simulink model "momentumBasedFlight"  (R2021b)
settings: Solver=VariableStepAuto  StartTime=0.0  StopTime=Config.simulationTime  RelTol=1e-3
InitFcn:
  | cd(fileparts(which(bdroot)));
  | initMomentumBasedFlight;
StopFcn:
  | cd(fileparts(which(bdroot)));
  | stopMomentumBasedFlight;
undefined symbols (not defined in the file or in its folder): aero_config, biasVectorConstraint_feet, Config, ConstraintMatrix_feet, DiscIntNeverNeededParam, frameNames, Frames
libraries: WBToolboxLibrary x104, momentum_flight_control_sublib x4, thrust_estimation_sublib x1, jets_control x1
(part 3 of 3)

== system momentumBasedFlight/FLIGHT CONTROLLER (CORE) V3.0/Flight Controller RAL-HUMANOIDS V3.0/Momentum Control for Flying/QP Solver and Integrate Contact Forces Derivative ==
  HessianMatrixQP : Inport
  gVectorQP : Inport  Port=2
  lowerBoundQP : Inport  Port=3
  upperBoundQP : Inport  Port=4
  stateMachineQuantities : Inport  Port=5
  systemState : Inport  Port=6
  dynamics : Inport  Port=7
  Bus Selector1 : BusSelector  OutputSignals=feetContactIsActive
  Bus Selector2 : BusSelector  OutputSignals=contactForces
  Integrate the Contact Forces Derivative : Subsystem
  QP momentumControl : Subsystem
  contactForces_star : Outport  VectorParamsAs1DForOutWhenUnconnected=off
  jetsIntensitiesDot_star : Outport  Port=2  VectorParamsAs1DForOutWhenUnconnected=off
  jointVel_star : Outport  Port=3  VectorParamsAs1DForOutWhenUnconnected=off
  tag scope: contactForces_star=global, exitFlagQP_momentumControl=global, jetsIntensitiesDot_star=global, jointVel_star=global
  wires:
  systemState/1 -> Bus Selector2/1
  Bus Selector2/1 -> Integrate the Contact Forces Derivative/2(contactForces)  "<contactForces>"
  Bus Selector1/1 -> Integrate the Contact Forces Derivative/4(feetContactIsActive), QP momentumControl/5(feetContactIsActive)  "<feetContactIsActive>"
  QP momentumControl/3(jointVel_star) -> jointVel_star/1, [jointVel_star]
  QP momentumControl/1(jetsIntensitiesDot_star) -> jetsIntensitiesDot_star/1, [jetsIntensitiesDot_star]
  HessianMatrixQP/1 -> QP momentumControl/1(HessianMatrixQP)
  stateMachineQuantities/1 -> Bus Selector1/1
  gVectorQP/1 -> QP momentumControl/2(gVectorQP)
  QP momentumControl/4(exitFlagQP_momentumControl) -> [exitFlagQP_momentumControl]
  upperBoundQP/1 -> QP momentumControl/4(upperBoundQP)
  lowerBoundQP/1 -> QP momentumControl/3(lowerBoundQP)
  Integrate the Contact Forces Derivative/1(contactForces_star) -> [contactForces_star], contactForces_star/1
  QP momentumControl/2(contactForcesDot_star) -> Integrate the Contact Forces Derivative/1(contactForcesDot_star)
  dynamics/1 -> Integrate the Contact Forces Derivative/3(dynamics)

== system momentumBasedFlight/FLOATING BASE ESTIMATOR/Compute base to fixed link transform/LFoot to base link transform /neck transform ==
  neck port : Inport
  Constant : Constant  Value=zeros(3,1)
  Gain : Gain  Gain=pi/180
  Selector1 : Selector  InputPortWidth=Ports.NECK_POS_PORT_SIZE  IndexOptions=Index vector (dialog)  Indices=[1:3]  OutputSizes=1
  Switch : Switch  Criteria=u2 > Threshold
  USE_IMU4EST_BASE1 : Constant  Value=Config.CORRECT_NECK_IMU
  neck position : Outport  VectorParamsAs1DForOutWhenUnconnected=off
  wires:
  neck port/1 -> Gain/1
  USE_IMU4EST_BASE1/1 -> Switch/2
  Switch/1 -> neck position/1
  Gain/1 -> Selector1/1
  Constant/1 -> Switch/3
  Selector1/1 -> Switch/1  "neck pos"

== system momentumBasedFlight/FLOATING BASE ESTIMATOR/Compute base to fixed link transform/RFoot to base link transform/neck transform ==
  neck port : Inport
  Constant : Constant  Value=zeros(3,1)
  Gain : Gain  Gain=pi/180
  Selector1 : Selector  InputPortWidth=Ports.NECK_POS_PORT_SIZE  IndexOptions=Index vector (dialog)  Indices=[1:3]  OutputSizes=1
  Switch : Switch  Criteria=u2 > Threshold
  USE_IMU4EST_BASE1 : Constant  Value=Config.CORRECT_NECK_IMU
  neck position : Outport  VectorParamsAs1DForOutWhenUnconnected=off
  wires:
  neck port/1 -> Gain/1
  USE_IMU4EST_BASE1/1 -> Switch/2
  Switch/1 -> neck position/1
  Gain/1 -> Selector1/1
  Constant/1 -> Switch/3
  Selector1/1 -> Switch/1  "neck pos"

== system momentumBasedFlight/FLIGHT CONTROLLER (CORE) V3.0/Flight Controller RAL-HUMANOIDS V3.0/Joint Torque Control for Flying/QP torqueControl/QP torqueControl - balancing ==
  H : Inport
  g : Inport  Port=2
  ub : Inport  Port=3
  lb : Inport  Port=4
  AEq : Inport  Port=5
  lbEq : Inport  Port=6
  ubEq : Inport  Port=7
  Enable : EnablePort
  Combine Bounds and Inequalities : MATLAB Function  TreatAsAtomicUnit=on
  MatchSignalSizes : WBToolboxLibrary/Utilities/MatchSignalSizes
      settings: SourceProductName=WholeBodyToolbox
  QP balancing-torqueControl : WBToolboxLibrary/Utilities/QP  lbA=on  ubA=on  lb=off  ub=off  computeObjVal=off  stopIfFails=off
      settings: SourceProductName=WholeBodyToolbox
  QPStatus_balancing : Outport  VectorParamsAs1DForOutWhenUnconnected=off
  QPOutput_balancing : Outport  Port=2  VectorParamsAs1DForOutWhenUnconnected=off
  wires:
  Combine Bounds and Inequalities/3(ubEq_combined) -> QP balancing-torqueControl/5
  Combine Bounds and Inequalities/2(lbEq_combined) -> QP balancing-torqueControl/4
  Combine Bounds and Inequalities/1(AEq_combined) -> QP balancing-torqueControl/3
  ub/1 -> Combine Bounds and Inequalities/5(ub)
  lb/1 -> Combine Bounds and Inequalities/4(lb)
  ubEq/1 -> Combine Bounds and Inequalities/3(ubEq)
  lbEq/1 -> Combine Bounds and Inequalities/2(lbEq)
  AEq/1 -> Combine Bounds and Inequalities/1(AEq)
  g/1 -> QP balancing-torqueControl/2, MatchSignalSizes/1
  H/1 -> QP balancing-torqueControl/1
  QP balancing-torqueControl/1 -> MatchSignalSizes/2
  MatchSignalSizes/1 -> QPOutput_balancing/1
  QP balancing-torqueControl/2 -> QPStatus_balancing/1

== system momentumBasedFlight/FLIGHT CONTROLLER (CORE) V3.0/Flight Controller RAL-HUMANOIDS V3.0/Joint Torque Control for Flying/QP torqueControl/QP torqueControl - flight ==
  H : Inport
  g : Inport  Port=2
  ub : Inport  Port=3
  lb : Inport  Port=4
  Enable : EnablePort
  Constant : Constant  Value=eye(Config.N_DOF)
  MatchSignalSizes : WBToolboxLibrary/Utilities/MatchSignalSizes
      settings: SourceProductName=WholeBodyToolbox
  QP flight-torqueControl : WBToolboxLibrary/Utilities/QP  lbA=on  ubA=on  lb=off  ub=off  computeObjVal=off  stopIfFails=off
      settings: SourceProductName=WholeBodyToolbox
  QPStatus_flight : Outport  VectorParamsAs1DForOutWhenUnconnected=off
  QPOutput_flight : Outport  Port=2  VectorParamsAs1DForOutWhenUnconnected=off
  wires:
  ub/1 -> QP flight-torqueControl/5
  g/1 -> MatchSignalSizes/1, QP flight-torqueControl/2
  H/1 -> QP flight-torqueControl/1
  QP flight-torqueControl/1 -> MatchSignalSizes/2
  MatchSignalSizes/1 -> QPOutput_flight/1
  lb/1 -> QP flight-torqueControl/4
  QP flight-torqueControl/2 -> QPStatus_flight/1
  Constant/1 -> QP flight-torqueControl/3

== system momentumBasedFlight/FLIGHT CONTROLLER (CORE) V3.0/Flight Controller RAL-HUMANOIDS V3.0/Joint Torque Control for Flying/QP torqueControl/Select QP torqueControl Output ==
  QPStatus_balancing : Inport
  QPOutput_balancing : Inport  Port=2
  feetContactIsActive : Inport  Port=3
  QPStatus_flight : Inport  Port=4
  QPOutput_flight : Inport  Port=5
  Demux : Demux  Outputs=[12;Config.N_DOF]
  Switch : Switch  Criteria=u2 > Threshold
  Switch1 : Switch  Criteria=u2 > Threshold
  jointTorques_star : Outport  VectorParamsAs1DForOutWhenUnconnected=off
  exitFlagQP_torqueControl : Outport  Port=2  VectorParamsAs1DForOutWhenUnconnected=off
  contactForces_QP_star : Outport  Port=3  VectorParamsAs1DForOutWhenUnconnected=off
  wires:
  Demux/2 -> Switch1/1
  Demux/1 -> contactForces_QP_star/1
  QPOutput_flight/1 -> Switch1/3
  QPOutput_balancing/1 -> Demux/1
  Switch/1 -> exitFlagQP_torqueControl/1
  QPStatus_flight/1 -> Switch/3
  QPStatus_balancing/1 -> Switch/1
  feetContactIsActive/1 -> Switch/2, Switch1/2
  Switch1/1 -> jointTorques_star/1

== system momentumBasedFlight/FLIGHT CONTROLLER (CORE) V3.0/Flight Controller RAL-HUMANOIDS V3.0/Momentum Control for Flying/QP Solver and Integrate Contact Forces Derivative/Integrate the Contact Forces Derivative ==
  contactForcesDot_star : Inport
  contactForces : Inport  Port=2
  dynamics : Inport  Port=3
  feetContactIsActive : Inport  Port=4
  Bus Selector2 : BusSelector  OutputSignals=M
  Discrete-Time Integrator1 : DiscreteIntegrator  ExternalReset=either  InitialConditionSource=external  InitialCondition=zeros(6,1)  SampleTime=Config.tStep  ICPrevOutput=DiscIntNeverNeededParam  ICPrevScaledInput=DiscIntNeverNeededParam
  Select Integrator Initial Condition : MATLAB Function  TreatAsAtomicUnit=on
  Selector : Selector  NumberOfDimensions=2  InputPortWidth=3  IndexOptions=Index vector (dialog),Index vector (dialog)  Indices=1,1  OutputSizes=1,1
  deadZone : Subsystem
  contactForces_star : Outport  VectorParamsAs1DForOutWhenUnconnected=off
  tag scope: contactForcesDot_star=global
  wires:
  Select Integrator Initial Condition/1(contactForces_0) -> Discrete-Time Integrator1/3
  feetContactIsActive/1 -> Discrete-Time Integrator1/2, Select Integrator Initial Condition/1(feetContactIsActive)
  contactForces/1 -> Select Integrator Initial Condition/2(contactForces)
  deadZone/1(u_cut) -> Discrete-Time Integrator1/1
  contactForcesDot_star/1 -> [contactForcesDot_star], deadZone/1(u)
  Discrete-Time Integrator1/1 -> contactForces_star/1
  dynamics/1 -> Bus Selector2/1
  Bus Selector2/1 -> Selector/1  "<M>"
  Selector/1 -> Select Integrator Initial Condition/3(m)

== system momentumBasedFlight/FLIGHT CONTROLLER (CORE) V3.0/Flight Controller RAL-HUMANOIDS V3.0/Momentum Control for Flying/QP Solver and Integrate Contact Forces Derivative/QP momentumControl ==
  HessianMatrixQP : Inport
  gVectorQP : Inport  Port=2
  lowerBoundQP : Inport  Port=3
  upperBoundQP : Inport  Port=4
  feetContactIsActive : Inport  Port=5
  NOT : Logic  Operator=NOT  IconShape=distinctive  AllPortsSameDT=off  OutDataTypeStr=boolean
  Process QP Inputs Momentum Control : MATLAB Function  TreatAsAtomicUnit=on
  QP momentumControl - balancing : Subsystem  TreatAsAtomicUnit=on
  QP momentumControl - flight : Subsystem  TreatAsAtomicUnit=on
  Select QP momentumControl Output : Subsystem
  jetsIntensitiesDot_star : Outport  VectorParamsAs1DForOutWhenUnconnected=off
  contactForcesDot_star : Outport  Port=2  VectorParamsAs1DForOutWhenUnconnected=off
  jointVel_star : Outport  Port=3  VectorParamsAs1DForOutWhenUnconnected=off
  exitFlagQP_momentumControl : Outport  Port=4  VectorParamsAs1DForOutWhenUnconnected=off
  wires:
  QP momentumControl - flight/2(QPOutput_flight) -> Select QP momentumControl Output/5(QPOutput_flight)
  QP momentumControl - flight/1(QPStatus_flight) -> Select QP momentumControl Output/4(QPStatus_flight)
  QP momentumControl - balancing/2(QPOutput_balancing) -> Select QP momentumControl Output/2(QPOutput_balancing)
  QP momentumControl - balancing/1(QPStatus_balancing) -> Select QP momentumControl Output/1(QPStatus_balancing)
  Select QP momentumControl Output/4(exitFlagQP_momentumControl) -> exitFlagQP_momentumControl/1
  NOT/1 -> QP momentumControl - flight/Enable
  Process QP Inputs Momentum Control/8(lb_flight) -> QP momentumControl - flight/4(lb)
  Process QP Inputs Momentum Control/7(ub_flight) -> QP momentumControl - flight/3(ub)
  Process QP Inputs Momentum Control/4(lb_balancing) -> QP momentumControl - balancing/4(lb)
  Process QP Inputs Momentum Control/3(ub_balancing) -> QP momentumControl - balancing/3(ub)
  Process QP Inputs Momentum Control/6(g_flight) -> QP momentumControl - flight/2(g)
  Process QP Inputs Momentum Control/5(H_flight) -> QP momentumControl - flight/1(H)
  Process QP Inputs Momentum Control/2(g_balancing) -> QP momentumControl - balancing/2(g)
  Process QP Inputs Momentum Control/1(H_balancing) -> QP momentumControl - balancing/1(H)
  Select QP momentumControl Output/2(contactForcesDot_star) -> contactForcesDot_star/1
  Select QP momentumControl Output/3(jointVel_star) -> jointVel_star/1
  Select QP momentumControl Output/1(jetsIntensitiesDot_star) -> jetsIntensitiesDot_star/1
  HessianMatrixQP/1 -> Process QP Inputs Momentum Control/1(HessianMatrixQP)
  upperBoundQP/1 -> Process QP Inputs Momentum Control/4(upperBoundQP)
  feetContactIsActive/1 -> QP momentumControl - balancing/Enable, NOT/1, Select QP momentumControl Output/3(feetContactIsActive)
  lowerBoundQP/1 -> Process QP Inputs Momentum Control/3(lowerBoundQP)
  gVectorQP/1 -> Process QP Inputs Momentum Control/2(gVectorQP)

== system momentumBasedFlight/FLIGHT CONTROLLER (CORE) V3.0/Flight Controller RAL-HUMANOIDS V3.0/Momentum Control for Flying/QP Solver and Integrate Contact Forces Derivative/Integrate the Contact Forces Derivative/deadZone ==
  u : Inport
  Constant : Constant  Value=Config.sat.deadZoneThreshold
  Deadzone Function : MATLAB Function  TreatAsAtomicUnit=on
  u_cut : Outport  VectorParamsAs1DForOutWhenUnconnected=off
  wires:
  Constant/1 -> Deadzone Function/2(thr)
  u/1 -> Deadzone Function/1(u)
  Deadzone Function/1(y) -> u_cut/1

== system momentumBasedFlight/FLIGHT CONTROLLER (CORE) V3.0/Flight Controller RAL-HUMANOIDS V3.0/Momentum Control for Flying/QP Solver and Integrate Contact Forces Derivative/QP momentumControl/QP momentumControl - balancing ==
  H : Inport
  g : Inport  Port=2
  ub : Inport  Port=3
  lb : Inport  Port=4
  Enable : EnablePort
  Constant : Constant  Value=eye(Config.N_DOF + 12 + 4)
  MatchSignalSizes : WBToolboxLibrary/Utilities/MatchSignalSizes
      settings: SourceProductName=WholeBodyToolbox
  QP : WBToolboxLibrary/Utilities/QP  lbA=on  ubA=on  lb=off  ub=off  computeObjVal=off  stopIfFails=off
      settings: SourceProductName=WholeBodyToolbox
  QPStatus_balancing : Outport  VectorParamsAs1DForOutWhenUnconnected=off
  QPOutput_balancing : Outport  Port=2  VectorParamsAs1DForOutWhenUnconnected=off
  wires:
  ub/1 -> QP/5
  QP/1 -> MatchSignalSizes/2
  MatchSignalSizes/1 -> QPOutput_balancing/1
  QP/2 -> QPStatus_balancing/1
  H/1 -> QP/1
  g/1 -> MatchSignalSizes/1, QP/2
  lb/1 -> QP/4
  Constant/1 -> QP/3

== system momentumBasedFlight/FLIGHT CONTROLLER (CORE) V3.0/Flight Controller RAL-HUMANOIDS V3.0/Momentum Control for Flying/QP Solver and Integrate Contact Forces Derivative/QP momentumControl/QP momentumControl - flight ==
  H : Inport
  g : Inport  Port=2
  ub : Inport  Port=3
  lb : Inport  Port=4
  Enable : EnablePort
  Constant : Constant  Value=eye(Config.N_DOF + 4)
  MatchSignalSizes : WBToolboxLibrary/Utilities/MatchSignalSizes
      settings: SourceProductName=WholeBodyToolbox
  QP flight-momentumControl : WBToolboxLibrary/Utilities/QP  lbA=on  ubA=on  lb=off  ub=off  computeObjVal=off  stopIfFails=off
      settings: SourceProductName=WholeBodyToolbox
  QPStatus_flight : Outport  VectorParamsAs1DForOutWhenUnconnected=off
  QPOutput_flight : Outport  Port=2  VectorParamsAs1DForOutWhenUnconnected=off
  wires:
  ub/1 -> QP flight-momentumControl/5
  g/1 -> MatchSignalSizes/1, QP flight-momentumControl/2
  H/1 -> QP flight-momentumControl/1
  QP flight-momentumControl/1 -> MatchSignalSizes/2
  MatchSignalSizes/1 -> QPOutput_flight/1
  lb/1 -> QP flight-momentumControl/4
  QP flight-momentumControl/2 -> QPStatus_flight/1
  Constant/1 -> QP flight-momentumControl/3

== system momentumBasedFlight/FLIGHT CONTROLLER (CORE) V3.0/Flight Controller RAL-HUMANOIDS V3.0/Momentum Control for Flying/QP Solver and Integrate Contact Forces Derivative/QP momentumControl/Select QP momentumControl Output ==
  QPStatus_balancing : Inport
  QPOutput_balancing : Inport  Port=2
  feetContactIsActive : Inport  Port=3
  QPStatus_flight : Inport  Port=4
  QPOutput_flight : Inport  Port=5
  Constant : Constant  Value=zeros(12,1)
  Demux : Demux  Outputs=[4;12;Config.N_DOF]
  Demux1 : Demux  Outputs=[4;Config.N_DOF]
  Switch{,1..3} (4 alike) : Switch  Criteria=u2 > Threshold
  jetsIntensitiesDot_star : Outport  VectorParamsAs1DForOutWhenUnconnected=off
  contactForcesDot_star : Outport  Port=2  VectorParamsAs1DForOutWhenUnconnected=off
  jointVel_star : Outport  Port=3  VectorParamsAs1DForOutWhenUnconnected=off
  exitFlagQP_momentumControl : Outport  Port=4  VectorParamsAs1DForOutWhenUnconnected=off
  wires:
  Demux1/2 -> Switch3/3
  Demux/3 -> Switch3/1
  Constant/1 -> Switch2/3
  Demux/2 -> Switch2/1
  Demux1/1 -> Switch1/3
  Demux/1 -> Switch1/1
  QPOutput_flight/1 -> Demux1/1
  QPOutput_balancing/1 -> Demux/1
  Switch/1 -> exitFlagQP_momentumControl/1
  QPStatus_flight/1 -> Switch/3
  QPStatus_balancing/1 -> Switch/1
  feetContactIsActive/1 -> Switch/2, Switch1/2, Switch2/2, Switch3/2
  Switch3/1 -> jointVel_star/1
  Switch1/1 -> jetsIntensitiesDot_star/1
  Switch2/1 -> contactForcesDot_star/1

== matlab function momentumBasedFlight/Visualizer/Task and Base Frame Kinematics/MATLAB Function3 ==
  data: RPY_Corr output; rollPitchYaw input
function RPY_Corr = correctYawAngleFCN(rollPitchYaw)

    RPY_Corr = correctYawAngle(rollPitchYaw);

end

== matlab function momentumBasedFlight/Visualizer/Task and Base Frame Kinematics/Get RPY from rotation matrix  ==
  data: w_R_b input; rollPitchYaw output
function rollPitchYaw = rollPitchYawFromRotationFCN(w_R_b)

rollPitchYaw = wbc.rollPitchYawFromRotation(w_R_b);

end

== matlab function momentumBasedFlight/FLIGHT CONTROLLER (CORE) V3.0/Estimated or Measured Thrusts/fromPosRPYtoTransfMatrix ==
  data: pos_rpy input; w_H_b output
function w_H_b = fromPosRpyToTransfMatrixFCN(pos_rpy)

    w_H_b = wbc.fromPosRpyToTransfMatrix(pos_rpy);
end

== matlab function momentumBasedFlight/Visualizer/Task and Base Frame Kinematics/Get RPY from rotation matrix ==
  data: w_R_b input; rollPitchYaw output
function rollPitchYaw = rollPitchYawFromRotationFCN(w_R_b)

rollPitchYaw = wbc.rollPitchYawFromRotation(w_R_b);

end

== matlab function momentumBasedFlight/Visualizer/Task and Base Frame Kinematics/Get RPY error norm ==
  data: rot_err input; rotErr_norm output
function rotErr_norm = normFCN(rot_err)

rotErr_norm = norm(rot_err);

end

== matlab function momentumBasedFlight/FLIGHT CONTROLLER (CORE) V3.0/Flight Controller RAL-HUMANOIDS V3.0/Joint Torque Control for Flying/QP torqueControl/Process QP Inputs Torque Control ==
  data: HessianMatrixQP input; H_balancing output; gVectorQP input; InequalityConstrMatrix input; biasVectorInequalityConstr input; g_balancing output; ub_balancing output; lb_balancing output; Aeq_balancing output; lbEq_balancing output; ubEq_balancing output; H_flight output; g_flight output; ub_flight output; lb_flight output; jointTorquesSaturation input; Config parameter
function [H_balancing,g_balancing,ub_balancing,lb_balancing,Aeq_balancing,lbEq_balancing,ubEq_balancing, ...
          H_flight,g_flight,ub_flight,lb_flight] = processQPinputTorqueControlFCN ...
                                                       (HessianMatrixQP,gVectorQP,InequalityConstrMatrix, ...
                                                        biasVectorInequalityConstr,jointTorquesSaturation,Config)   
   
[H_balancing,g_balancing,ub_balancing,lb_balancing,Aeq_balancing,lbEq_balancing,ubEq_balancing, ...
          H_flight,g_flight,ub_flight,lb_flight] = iRonCubLib.processQPinputTorqueControl ...
                                                       (HessianMatrixQP,gVectorQP,InequalityConstrMatrix, ...
                                                        biasVectorInequalityConstr,jointTorquesSaturation,Config);     
end

== matlab function momentumBasedFlight/FLIGHT CONTROLLER (CORE) V3.0/Flight Controller RAL-HUMANOIDS V3.0/Joint Torque Control for Flying/QP torqueControl/QP torqueControl - balancing/Combine Bounds and Inequalities ==
  data: AEq input; AEq_combined output; lbEq input; ubEq input; lb input; ub input; lbEq_combined output; ubEq_combined output
function [AEq_combined,lbEq_combined,ubEq_combined] = combineInputBoundsAndInequalitiesQPFCN(AEq,lbEq,ubEq,lb,ub)

   [AEq_combined,lbEq_combined,ubEq_combined] = iRonCubLib.combineInputBoundsAndInequalitiesQP(AEq,lbEq,ubEq,lb,ub);
end

== matlab function momentumBasedFlight/Visualizer/Task and Base Frame Kinematics/MATLAB Function2 ==
  data: RPY_Corr output; rollPitchYaw input
function RPY_Corr = correctYawAngleFCN(rollPitchYaw)

    RPY_Corr = correctYawAngle(rollPitchYaw);

end

== matlab function momentumBasedFlight/FLIGHT CONTROLLER (CORE) V3.0/Flight Controller RAL-HUMANOIDS V3.0/Joint Torque Control for Flying/Torque Derivative Saturation/Saturate Torque Derivative ==
  data: u input; uSat output; u_0 input; tStep input; uDotMax input
function uSat = saturateInputDerivativeFCN(u, u_0, tStep, uDotMax)

    uSat = wbc.saturateInputDerivative(u, u_0, tStep, uDotMax);
end

== matlab function momentumBasedFlight/FLIGHT CONTROLLER (CORE) V3.0/Flight Controller RAL-HUMANOIDS V3.0/Joint Torque Control for Flying/torqueControlFCN ==
  data: M input; h input; J_jets input; J_LFoot input; J_RFoot input; JDot_LFoot_nu input; JDot_RFoot_nu input; J_aeroForces input; w_H_LFoot input; w_H_RFoot input; matrixOfJetsAxes input; ConstraintsMatrix_feet input; biasVectorConstraint_feet input; jetsIntensities input; stateVel input; jointVel_star input; contactForces_star input; KI_torqueControl input; KP_torqueControl input; feetContactIsActive input; activateEqConstrTorqueControl input; robotIsLanded input; aerodynamic_forces input; jointPos_err input; Hessian output; Config parameter; gradient output; ConstraintMatrix_inequality output; biasVectorConstraint_inequality output; jointVel_err output; sDDot_star output; aero_config parameter; St_invM_B output; St_invM_bias output
function [Hessian, gradient, ConstraintMatrix_inequality, biasVectorConstraint_inequality, jointVel_err,sDDot_star, St_invM_B, St_invM_bias] =  ... 
             aeroFlyingTorqueControlFCN(M, h, J_jets, J_LFoot, J_RFoot, JDot_LFoot_nu, JDot_RFoot_nu, J_aeroForces, w_H_LFoot, w_H_RFoot, matrixOfJetsAxes, ...
                                        ConstraintsMatrix_feet, biasVectorConstraint_feet, jetsIntensities, stateVel, jointVel_star, contactForces_star, ...
                                        KI_torqueControl, KP_torqueControl, feetContactIsActive, activateEqConstrTorqueControl, robotIsLanded, aerodynamic_forces, jointPos_err, Config, aero_config)
                                      
    [Hessian, gradient, ConstraintMatrix_inequality, biasVectorConstraint_inequality, jointVel_err,sDDot_star, St_invM_B, St_invM_bias] =  ... 
        aeroFlyingTorqueControl(M, h, J_jets, J_LFoot, J_RFoot, JDot_LFoot_nu, JDot_RFoot_nu, J_aeroForces, w_H_LFoot, w_H_RFoot, matrixOfJetsAxes, ...
                                ConstraintsMatrix_feet, biasVectorConstraint_feet, jetsIntensities, stateVel, jointVel_star, contactForces_star, ...
                                KI_torqueControl, KP_torqueControl, feetContactIsActive, activateEqConstrTorqueControl, robotIsLanded, aerodynamic_forces, jointPos_err, aero_config, Config);           
end

== matlab function momentumBasedFlight/FLIGHT CONTROLLER (CORE) V3.0/Flight Controller RAL-HUMANOIDS V3.0/Momentum Control for Flying/Momentum Control/Aerodynamic Flying Controller Momentum FCN  ==
  data: jointPos input; w_baseTwist input; jetsIntensities input; J_jets input; J_CoM input; J_LFoot input; J_RFoot input; posCoM input; w_R_b input; w_H_LFoot input; w_H_RFoot input; matrixOfJetsAxes input; matrixOfJetsArms input; matrixOfAeroArms input; J_aeroForces input; w_I_c input; L input; M input; CMM input; pos_vel_acc_jerk_CoM_des input; rot_vel_acc_jerk_base_des input size=[3,6]; jointPos_des input; KP_momentum input; KD_momentum input; KP_postural input; feetContactIsActive input; decreaseMaxFootVerticalForce input; increaseMinFootVerticalForce input; robotIsLanded input; HessianMatrixQP output; gVectorQP output; lowerBoundQP output; upperBoundQP output; L_des output; LDot_estimated output; verifyAngMomAndInertia output; contactForces_hat input; aerodynamic_forces input; Config parameter; velCoM output; aero_config parameter
function [HessianMatrixQP, gVectorQP, lowerBoundQP, upperBoundQP, L_des, LDot_estimated, verifyAngMomAndInertia, velCoM] = ...
             aeroFlyingMomentumControlFCN(jointPos, w_baseTwist, jetsIntensities, J_jets, J_CoM, J_LFoot, J_RFoot, posCoM, w_R_b, w_H_LFoot, w_H_RFoot, ...
                                          matrixOfJetsAxes, matrixOfJetsArms, matrixOfAeroArms, J_aeroForces, w_I_c, L, M, CMM, pos_vel_acc_jerk_CoM_des, ....
                                          rot_vel_acc_jerk_base_des, jointPos_des, KP_momentum, KD_momentum, KP_postural, feetContactIsActive, ...
                                          decreaseMaxFootVerticalForce, increaseMinFootVerticalForce, robotIsLanded, contactForces_hat, aerodynamic_forces, Config, aero_config)
                               
    [HessianMatrixQP, gVectorQP, lowerBoundQP, upperBoundQP, L_des, LDot_estimated, verifyAngMomAndInertia, velCoM] = ...
        aeroFlyingMomentumControl(jointPos, w_baseTwist, jetsIntensities, J_jets, J_CoM, J_LFoot, J_RFoot, posCoM, w_R_b, w_H_LFoot, w_H_RFoot, ...
                                  matrixOfJetsAxes, matrixOfJetsArms, matrixOfAeroArms, J_aeroForces, w_I_c, L, M, CMM, pos_vel_acc_jerk_CoM_des, ....
                                  rot_vel_acc_jerk_base_des, jointPos_des, KP_momentum, KD_momentum, KP_postural, feetContactIsActive, ...
                                  decreaseMaxFootVerticalForce, increaseMinFootVerticalForce, robotIsLanded, contactForces_hat, aerodynamic_forces, aero_config, Config);
end

== matlab function momentumBasedFlight/FLIGHT CONTROLLER (CORE) V3.0/Flight Controller RAL-HUMANOIDS V3.0/Momentum Control for Flying/QP Solver and Integrate Contact Forces Derivative/Integrate the Contact Forces Derivative/Select Integrator Initial Condition ==
  data: feetContactIsActive input; contactForces input; contactForces_0 output; m input; Config parameter
function contactForces_0 = selectInitContactForces_noFT_FCN(feetContactIsActive, contactForces, m, Config)

    contactForces_0 = selectInitContactForces_noFT(feetContactIsActive, contactForces, m, Config);
end

== matlab function momentumBasedFlight/FLIGHT CONTROLLER (CORE) V3.0/Dynamics and Kinematics/Kinematic Quantities/Compute Aerodynamic Forces Arms/Thrust Axes and Arms ==
  data: w_H_LinkFrames input; posCoM input; matrixOfAeroArms output; Config parameter; aero_config parameter
function matrixOfAeroArms = computeAeroArmsFCN(w_H_LinkFrames, posCoM, Config, aero_config)

    matrixOfAeroArms = computeAeroArms(w_H_LinkFrames, posCoM, aero_config, Config);
end

== matlab function momentumBasedFlight/FLIGHT CONTROLLER (CORE) V3.0/Dynamics and Kinematics/Kinematic Quantities/Compute Aerodynamic Forces Homogeneous Transform/Aero Transforms ==
  data: w_H_LinkFrames input; posCoM input; matrixOfLinkCoMTransform output; Config parameter; aero_config parameter
function matrixOfLinkCoMTransform = computeMatrixOfLinkCoMTransformFCN(w_H_LinkFrames, posCoM, Config, aero_config)

    matrixOfLinkCoMTransform = computeMatrixOfLinkCoMTransform(w_H_LinkFrames, posCoM, aero_config, Config);
end

== matlab function momentumBasedFlight/FLIGHT CONTROLLER (CORE) V3.0/UpdateGuiData/Update Data for the GUI ==
  data: time input
function updateVisualGuiFCN(time)

    coder.extrinsic('updateVisualGui')

    persistent updateTime

    % for now I hard-coded 0.25 [s] as updating time for the data GUI
    timeStepGui    = 0.25;

    if isempty(updateTime)
    
        updateTime = timeStepGui;
    end
    
    % update data GUI
    if time > updateTime
    
        updateVisualGui;
        updateTime = time + timeStepGui;  
    end
end

== matlab function momentumBasedFlight/FLOATING BASE ESTIMATOR/Compute base to fixed link transform/LFoot to base link transform /Get Base Rotation From IMU ==
  data: imu_H_fixedLink input; imu_H_fixedLink_0 input; fixedLink_H_base input; rpyFromIMU_0 input; rpyFromIMU input; neck_pos input; w_H_b output; Config parameter
function w_H_b = getWorldToBaseTransformFCN(imu_H_fixedLink, imu_H_fixedLink_0, fixedLink_H_base, rpyFromIMU_0, rpyFromIMU, neck_pos, Config)

    FILTER_IMU_YAW = Config.FILTER_IMU_YAW;
    
    [w_H_b, wImu_H_base, wImu_H_fixedLink_0] = wbc.worldToBaseTransformWithIMU(imu_H_fixedLink, imu_H_fixedLink_0, fixedLink_H_base, rpyFromIMU_0, rpyFromIMU, FILTER_IMU_YAW);
    
    % Correct head IMU with neck positions (HEAD IMU only)
    if Config.CORRECT_NECK_IMU
        
        wImu_H_wImuAssumingNeckToZero = wbc.correctIMUWithNeckPos(neck_pos);
        wImu_H_base                   = wImu_H_wImuAssumingNeckToZero * wImu_H_base;
        w_H_b                         = wImu_H_fixedLink_0\wImu_H_base;  
    end
end

== matlab function momentumBasedFlight/FLIGHT CONTROLLER (CORE) V3.0/Dynamics and Kinematics/Dynamic Quantities/Compute Centroidal Inertia/Compute Centroidal Inertia ==
  data: M input; w_I_c output; posCoM input; posBase input
function w_I_c = getCentrInertiaFCN(M, posCoM, posBase)

    w_I_c = iRonCubLib.getCentrInertia(M, posCoM, posBase);
end

== matlab function momentumBasedFlight/FLIGHT CONTROLLER (CORE) V3.0/Dynamics and Kinematics/Kinematic Quantities/Compute Thrusts Axes and Arms/Thrust Axes and Arms ==
  data: w_H_J1 input; matrixOfJetsAxes output; w_H_J2 input; w_H_J3 input; w_H_J4 input; posCoM input; matrixOfJetsArms output; Config parameter
function [matrixOfJetsAxes, matrixOfJetsArms] = computeJetsAxesAndArmsFCN(w_H_J1, w_H_J2, w_H_J3, w_H_J4, posCoM, Config)

    [matrixOfJetsAxes, matrixOfJetsArms] = iRonCubLib.computeJetsAxesAndArms(w_H_J1, w_H_J2, w_H_J3, w_H_J4, posCoM, Config);
end

== matlab function momentumBasedFlight/FLIGHT CONTROLLER (CORE) V3.0/Dynamics and Kinematics/Kinematic Quantities/Compute Aerodynamic Forces Jacobians/compute matrix of link CoM Jacobians ==
  data: w_H_b input; linkFrameJacobians input; J_aeroForces output; aero_config parameter
function J_aeroForces = computeMatrixOfLinkCoMJacobians(w_H_b, linkFrameJacobians, aero_config)

    J_aeroForces = computeMatrixOfLinkCoMJacobians(w_H_b, linkFrameJacobians, aero_config);

end

== matlab function momentumBasedFlight/FLOATING BASE ESTIMATOR/Compute base to fixed link transform/RFoot to base link transform/Get Base Rotation From IMU ==
  data: imu_H_fixedLink input; imu_H_fixedLink_0 input; fixedLink_H_base input; rpyFromIMU_0 input; rpyFromIMU input; neck_pos input; w_H_b output; Config parameter
function w_H_b = getWorldToBaseTransformFCN(imu_H_fixedLink, imu_H_fixedLink_0, fixedLink_H_base, rpyFromIMU_0, rpyFromIMU, neck_pos, Config)

    FILTER_IMU_YAW = Config.FILTER_IMU_YAW;
    
    [w_H_b, wImu_H_base, wImu_H_fixedLink_0] = wbc.worldToBaseTransformWithIMU(imu_H_fixedLink, imu_H_fixedLink_0, fixedLink_H_base, rpyFromIMU_0, rpyFromIMU, FILTER_IMU_YAW);
    
    % Correct head IMU with neck positions (HEAD IMU only)
    if Config.CORRECT_NECK_IMU
        
        wImu_H_wImuAssumingNeckToZero = wbc.correctIMUWithNeckPos(neck_pos);
        wImu_H_base                   = wImu_H_wImuAssumingNeckToZero * wImu_H_base;
        w_H_b                         = wImu_H_fixedLink_0\wImu_H_base;  
    end
end

== matlab function momentumBasedFlight/FLIGHT CONTROLLER (CORE) V3.0/Generate wind profile/MATLAB Function ==
  data: maxWindSpeed input; windSpeed output; time input
function windSpeed = generatewindSpeed(maxWindSpeed, time)
    
    time_windStart = 10;
    time_maxWind   = 15;
    
    if time <= time_windStart
        windSpeed = zeros(3,1);
    else 
        if (time > time_windStart && time <= time_maxWind)
            windSpeed = maxWindSpeed * (time - time_windStart)/(time_maxWind - time_windStart);
        else
            windSpeed = maxWindSpeed;
        end
    end

end

== matlab function momentumBasedFlight/FLOATING BASE ESTIMATOR/Compute State Velocity/Compute Base Velocity ==
  data: J_l_sole input; J_r_sole input; feetContactStatus input; nu_b output; jointVel input; Reg parameter
function nu_b = computeBaseVelocityFCN(J_l_sole, J_r_sole, feetContactStatus, jointVel, Reg)

    pinvDamp_baseVel = Reg.pinvDamp_baseVel;
    
    nu_b = wbc.computeBaseVelocityWithFeetContact(J_l_sole, J_r_sole, feetContactStatus, jointVel, pinvDamp_baseVel);
end

== matlab function momentumBasedFlight/FLOATING BASE ESTIMATOR/baseState_feetFixed ==
  data: nu input; w_H_b_yoga input; outBaseState output
function outBaseState = calculateBaseEst(nu, w_H_b_yoga)

outBaseState        = zeros(18,1);
outBaseState(1:3)   = w_H_b_yoga(1:3,4);
outBaseState(4:6)   = wbc.rollPitchYawFromRotation(w_H_b_yoga(1:3,1:3));
outBaseState(7:12)  = nu(1:6);
end

== matlab function momentumBasedFlight/FLIGHT CONTROLLER (CORE) V3.0/Flight Controller RAL-HUMANOIDS V3.0/Joint Torque Control for Flying/Plot Torque QP Residuals/MATLAB Function ==
  data: jointTorques_star input; contactForces_QP_star input; residual_sDDot output; sDDot_star input; St_invM_B input; St_invM_bias input
function residual_sDDot = fcn(jointTorques_star, contactForces_QP_star, sDDot_star, St_invM_B, St_invM_bias)

residual_sDDot = St_invM_B*[contactForces_QP_star; jointTorques_star] + St_invM_bias - sDDot_star;

== matlab function momentumBasedFlight/FLIGHT CONTROLLER (CORE) V3.0/Flight Controller RAL-HUMANOIDS V3.0/Momentum Control for Flying/QP Solver and Integrate Contact Forces Derivative/Integrate the Contact Forces Derivative/deadZone/Deadzone Function ==
  data: u input; y output; thr input
function y = deadZoneFCN(u, thr)

    y = wbc.deadZone(u, thr);
end

== matlab function momentumBasedFlight/FLIGHT CONTROLLER (CORE) V3.0/Flight Controller RAL-HUMANOIDS V3.0/Momentum Control for Flying/QP Solver and Integrate Contact Forces Derivative/QP momentumControl/Process QP Inputs Momentum Control ==
  data: HessianMatrixQP input; H_balancing output; gVectorQP input; lowerBoundQP input; upperBoundQP input; g_balancing output; ub_balancing output; lb_balancing output; H_flight output; g_flight output; ub_flight output; lb_flight output
function [H_balancing,g_balancing,ub_balancing,lb_balancing, ...
          H_flight,g_flight,ub_flight,lb_flight] = processQPinputMomentumControlFCN(HessianMatrixQP,gVectorQP,lowerBoundQP,upperBoundQP) 
      
    [H_balancing,g_balancing,ub_balancing,lb_balancing, ...
        H_flight,g_flight,ub_flight,lb_flight] = iRonCubLib.processQPinputMomentumControl(HessianMatrixQP,gVectorQP,lowerBoundQP,upperBoundQP);
end

== matlab function momentumBasedFlight/Visualizer/Task and Base Frame Kinematics/MATLAB Function1 ==
  data: RPY_Corr output; rollPitchYaw input
function RPY_Corr = correctYawAngleFCN(rollPitchYaw)

    RPY_Corr = correctYawAngle(rollPitchYaw);

end

== matlab function momentumBasedFlight/FLIGHT CONTROLLER (CORE) V3.0/Flight Controller RAL-HUMANOIDS V3.0/deadZone/Deadzone Function ==
  data: u input; y output; thr input
function y = deadZoneFCN(u, thr)

    y = wbc.deadZone(u, thr);
end
